simulink model "SkyHookModel_sim"  (R2024b)
settings: Solver=FixedStepAuto  StartTime=0.0  StopTime=inf  FixedStep=0.001  RelTol=1e-3
values from neighbouring files (symbols this model uses):
  A = [      0             1            0         0 ... (first row only)    [EstimateDamping.m]    (also in QuarterCarModel.m)
  A_Nodamp = [      0             1            0         0 ... (first row only)    [QuarterCarModel.m]
  B = [0; k1/m1; 0; 0]    [EstimateDamping.m]    (also in QuarterCarModel.m = [  0     0     0)
  C = [0, 0, 1, 0]    [EstimateDamping.m]    (also in QuarterCarModel.m = [1 0 0 0)
  D = 0    [EstimateDamping.m]    (also in QuarterCarModel.m = zeros(4,3))
libraries: simulink x1, dspxfrm3 x1, dspsrcs4 x1
settings Model: Creator=elija  LastModifiedBy=elija

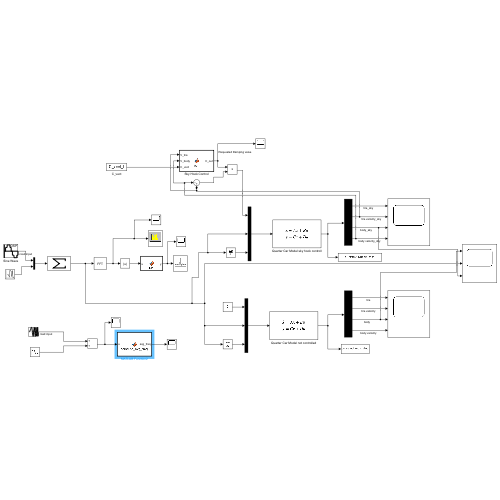
[thumbnail: Simulink's stored preview of the top-level diagram]
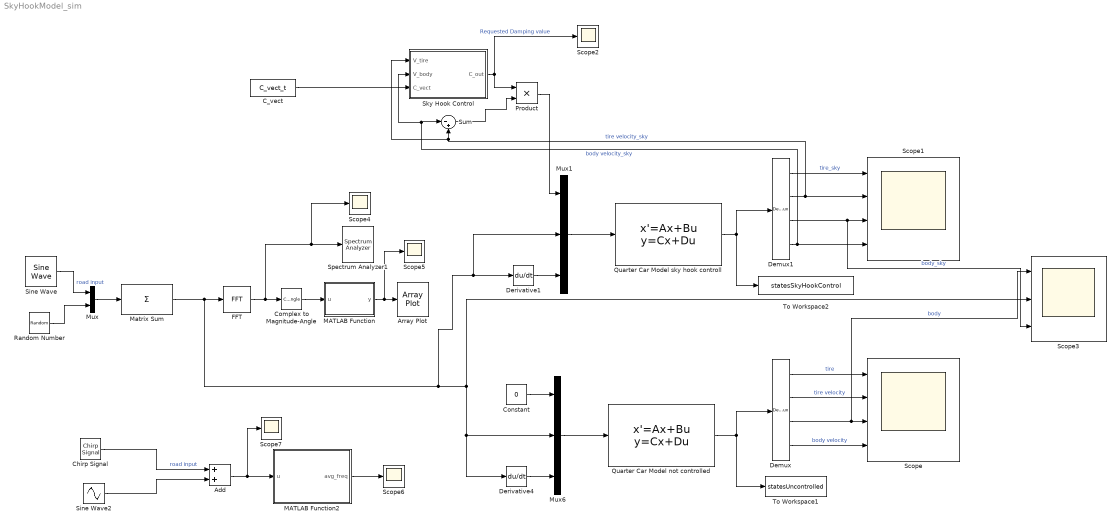
== system SkyHookModel_sim ==
  Add : Sum
  Array Plot : ArrayPlot  WindowPosition=[385.000000,40.000000,766.000000,784.000000,]  ScopeFrameLocation=window  MaximizeAxes=Off  YLimits=[1.692 2.1754]
  C_vect : FromWorkspace  VariableName=C_vect_t
  Chirp Signal : simulink/Sources/Chirp Signal  f1=0.1  T=20  f2=50
  Complex to Magnitude-Angle : ComplexToMagnitudeAngle  Output=Magnitude
  Constant : Constant  Value=0
  Demux : Demux
  Demux1 : Demux
  Derivative1 : Derivative
  Derivative4 : Derivative
  FFT : dspxfrm3/FFT  FFTImplementation=Auto  CompMethod=Table lookup  TableOpt=NEW  TableOptActive=Speed  BitRevOrder=off  Normalize=off  InheritFFTLength=on  FFTLength=64  WrapInput=on  roundingMode=Ceiling  overflowMode=off  firstCoeffDataTypeStr=Inherit: Same word length as input  firstCoeffLastDataTypeStr=Inherit: Same word length as input  outputMin=[]  outputMax=[]
  MATLAB Function : MATLAB Function  TreatAsAtomicUnit=on
  MATLAB Function2 : MATLAB Function  TreatAsAtomicUnit=on
  Matrix Sum : Sum  Inputs=+  CollapseMode=Specified dimension  CollapseDim=2
  Mux : Mux  Inputs=2
  Mux1 : Mux  Inputs=3
  Mux6 : Mux  Inputs=3
  Product : Product
  Quarter Car Model not controlled : StateSpace  A=A  B=B  C=C  D=D  InitialCondition=0
  Quarter Car Model sky hook controll : StateSpace  A=A_Nodamp  B=B  C=C  D=D  InitialCondition=0
  Random Number : RandomNumber  Variance=10  SampleTime=2
  Scope : Scope  NumInputPorts=4
  Scope1 : Scope  NumInputPorts=4
  Scope{2,4..7} (5 alike) : Scope
  Scope3 : Scope  NumInputPorts=3
  Sine Wave : dspsrcs4/Sine Wave  Amplitude=0.2  Frequency=[2 3 1 20 ]  Phase=0  SampleMode=Discrete  OutComplex=Real  CompMethod=Trigonometric fcn  TableSize=Speed  SampleTime=1/1000  SamplesPerFrame=1  ResetState=Restart at time zero  OutputFrames=off  dataType=double  wordLen=16  udDataType=sfix(16)  fracBitsMode=Best precision  numFracBits=15  OutDataTypeStr=double  LastOutDataTypeStr=double
  Sine Wave2 : Sin  Amplitude=0.01  Frequency=3  SampleTime=0
  Sky Hook Control : MATLAB Function  TreatAsAtomicUnit=on
  Spectrum Analyzer1 : SpectrumAnalyzer  WindowPosition=[368.000000,182.000000,800.000000,500.000000,]  ScopeFrameLocation=window  SpectrumType=Power density  Method=Welch  PlotAsTwoSidedSpectrum=off  AveragingMethod=Exponential  SpectrumUnits=dBm/Hz  YLimits=[-32.22475232,49.56111478]
  Sum : Sum  Inputs=|-+
  To Workspace1 : ToWorkspace  VariableName=statesUncontrolled  SaveFormat=Timeseries  SampleTime=-1
  To Workspace2 : ToWorkspace  VariableName=statesSkyHookControl  SaveFormat=Timeseries  SampleTime=-1
  wires:
  Constant/1 -> Mux6/1
  Mux6/1 -> Quarter Car Model not controlled/1
  Derivative4/1 -> Mux6/3
  Quarter Car Model not controlled/1 -> Demux/1, To Workspace1/1
  Demux/1 -> Scope/1  "tire"
  Demux/2 -> Scope/2  "tire velocity"
  Demux/3 -> Scope3/1, Scope/3  "body"
  Demux/4 -> Scope/4  "body velocity"
  Demux1/2 -> Scope1/2, Sky Hook Control/1(V_tire), Sum/2  "tire velocity_sky"
  Demux1/4 -> Scope1/4, Sky Hook Control/2(V_body), Sum/1  "body velocity_sky"
  Mux1/1 -> Quarter Car Model sky hook controll/1
  Derivative1/1 -> Mux1/3
  Quarter Car Model sky hook controll/1 -> Demux1/1, To Workspace2/1
  Demux1/3 -> Scope3/3, Scope1/3  "body_sky"
  Sine Wave/1 -> Mux/1  "road input"
  Demux1/1 -> Scope1/1  "tire_sky"
  Sum/1 -> Product/2
  C_vect/1 -> Sky Hook Control/3(C_vect)
  Product/1 -> Mux1/1
  Sky Hook Control/1(C_out) -> Product/1, Scope2/1  "Requested Damping value"
  Matrix Sum/1 -> Mux1/2, Derivative1/1, Scope3/2, Derivative4/1, Mux6/2, FFT/1
  FFT/1 -> Spectrum Analyzer1/1, Scope4/1, Complex to Magnitude-Angle/1
  MATLAB Function/1(y) -> Scope5/1, Array Plot/1
  Complex to Magnitude-Angle/1 -> MATLAB Function/1(u)
  Random Number/1 -> Mux/2
  Mux/1 -> Matrix Sum/1
  MATLAB Function2/1(avg_freq) -> Scope6/1
  Sine Wave2/1 -> Add/2
  Chirp Signal/1 -> Add/1  "road input"
  Add/1 -> Scope7/1, MATLAB Function2/1(u)

== matlab function SkyHookModel_sim/MATLAB Function ==
  data: u input; y output
function y = fcn(u)

y = fftshift(u);

== matlab function SkyHookModel_sim/Sky Hook Control ==
  settings: updateMethod=DISCRETE  sampleTime=0.001
  data: V_tire input; C_out output; V_body input; C_vect input
function C_out = fcn( V_tire, V_body, C_vect)
dC = 2;
    persistent C_prev  % Store previous value of C_out
    
    if isempty(C_prev)
        C_prev = C_vect(2); % Initialize with C_min
    end

    C_max = C_vect(1);
    C_min = C_vect(2);

    % Determine target value based on condition
    if -V_tire * (V_tire - V_body) > 0
        C_target = C_max;
    else
        C_target = C_min;
    end

    % Increment or decrement linearly towards target
    if C_prev < C_target
        C_out = min(C_prev + dC, C_target); % Move up with step dC
    elseif C_prev > C_target
        C_out = max(C_prev - dC, C_target); % Move down with step dC
    else
        C_out = C_prev; % Stay at the target if reached
    end

    % Store updated value for next function call
    C_prev = C_out;
end

% function C_out = fcn(V_tire, V_body, C_vect)
% 
% 
% C_max = C_vect(1);
% 
% C_min = C_vect(2);
% 
% if -V_tire.*(V_tire-V_body)>0
%     C_desired = C_max;
% 
% else
%     C_desired = C_min;   
% end
% 
% C_out = C_desired;
% 
% 
% 
% 
% end

== matlab function SkyHookModel_sim/MATLAB Function2 ==
  settings: updateMethod=DISCRETE
  data: u input; avg_freq output
function avg_freq = compute_avg_freq(u)

persistent buffer index Fs N last_avg_freq;

Fs = 1000;  % Sampling frequency (Hz)
N = 500;   % Window is 0.5 seconds. 

avg_freq = 0.0;  

if isempty(buffer)
    buffer = zeros(N, 1);
    index = 1;
    last_avg_freq = 0;
end

buffer(index) = u;
index = index + 1;
if index > N
    index = 1;
end

if index < N  
    avg_freq = last_avg_freq;  
    return;  
end

% Apply Hann window to reduce spectral leakage
window = hann(N);
Y = fft(buffer .* window);  
P2 = abs(Y) / sum(window);  
P1 = P2(1:N/2+1);  
P1(2:end-1) = 2 * P1(2:end-1);  
f = (0:(N/2)) * (Fs / N);  

% Find dominant frequency
[~, peak_idx] = max(P1);
peak_freq = f(min(peak_idx, length(f))); 


if isnan(peak_freq) || isinf(peak_freq)
    peak_freq = 0.0;
end
coder.extrinsic('disp');
disp(['Detected Frequency: ', sprintf('%.2f', peak_freq)]);
% disp(P1)
last_avg_freq = peak_freq*6.2; % not sure why we are off by a factor of 6.25
avg_freq = double(last_avg_freq);
